simulink model "Sim_Riementrieb_2015a"  (R2015a)
settings: Solver=ode45  SolverMode=SingleTasking  StartTime=0.0  StopTime=20.0  RelTol=1e-3
InitFcn:
  | set_parameter
libraries: cstblocks x2
settings Model: Creator=wke  LastModifiedBy=Andreas
settings DataIOCC: SignalLoggingSaveFormat=ModelDataLogs
settings OptimizationCC: BlockReduction=off  BooleanDataType=off
settings DebuggingCC: SaveWithParameterizedLinksMsg=none  UnderspecifiedInitializationDetection=Classic  MergeDetectMultiDrivingBlocksExec=none  SignalResolutionControl=TryResolveAllWithWarning  MultiTaskDSMMsg=warning  MultiTaskCondExecSysMsg=none  StateNameClashWarn=warning
settings HardwareCC: TargetUnknown=on

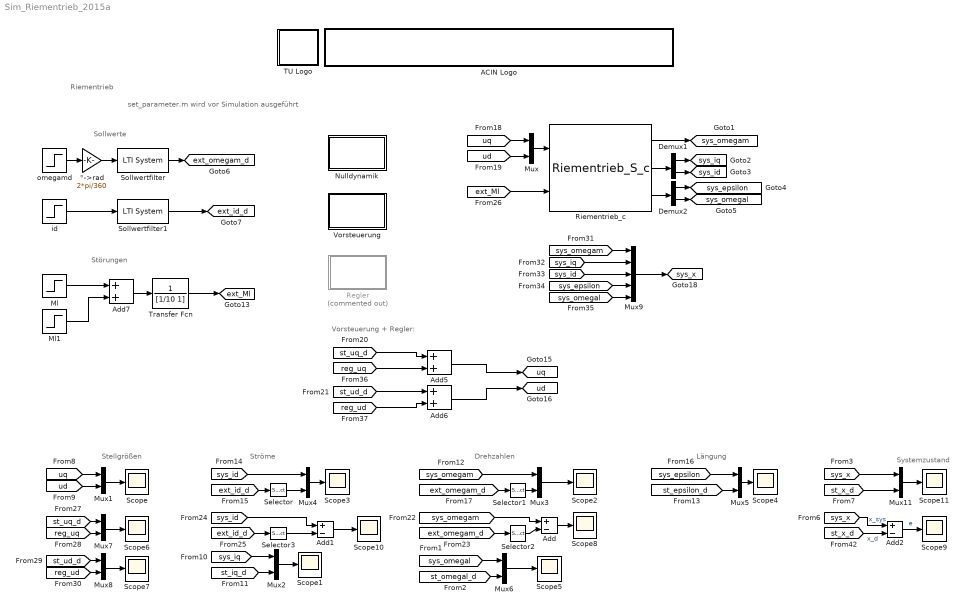
== system Sim_Riementrieb_2015a ==
  note: Vorsteuerung + Regler:
  note: Riementrieb
  note: set_parameter.m wird vor Simulation ausgeführt
  note: Sollwerte
  note: Stellgrößen
  note: Ströme
  note: Drehzahlen
  note: Längung
  note: Störungen
  note: Systemzustand
  ACIN Logo : Subsystem
      mask init:
      | s = get_param(gcb,'UserData');
      mask Display:
      | image(s.logo,[0 0 439 45]);
      | %axis image
  Add : Sum  Inputs=+-
  Add1 : Sum  Inputs=+-
  Add2 : Sum  Inputs=+-
  Add5 : Sum
  Add6 : Sum
  Add7 : Sum
  Demux1 : Demux  Outputs=2
  Demux2 : Demux  Outputs=2
  Ml : Step  Time=8  After=0.1  SampleTime=0
  Ml1 : Step  Time=15  After=-0.1  SampleTime=0
  Mux{,1..8,11} (10 alike) : Mux  Inputs=2
  Mux9 : Mux  Inputs=5
  Nulldynamik : Subsystem
  Regler : Subsystem  Commented=on
  Riementrieb_c : S-Function  FunctionName=Riementrieb_S_c  Parameters=parSys  SFunctionDeploymentMode=off  EnableBusSupport=off
      mask Display:
      | port_label('input',1,'uq,ud');
      | port_label('input',2,'Ml');
      | port_label('output',1,'omegam');
      | port_label('output',2,'iq,id');
      | port_label('output',3,'epsilon,omegal');
  Scope{,1..11} (12 alike) : Scope
      Scope settings: TimeRange=auto  ShowLegends=on  MaxDataPoints=5000  SaveToWorkspace=off  SaveName=ScopeData  YMin=3.34867  YMax=18.57408  SampleTime=-1
      Scope1 settings: TimeRange=auto  MaxDataPoints=5000  SaveToWorkspace=off  YMin=-300000  YMax=275000  SampleTime=-1
      Scope10 settings: TimeRange=auto  MaxDataPoints=5000  SaveToWorkspace=off  SaveName=ScopeData10  YMin=-10  YMax=10  SampleTime=-1
      Scope11 settings: TimeRange=auto  ShowLegends=on  MaxDataPoints=5000  SaveToWorkspace=off  SaveName=ScopeData11  YMin=-13.18283  YMax=118.51223  SampleTime=-1
      Scope2 settings: TimeRange=0.3051681706316654  ShowLegends=on  MaxDataPoints=5000  SaveToWorkspace=off  SaveName=ScopeData2  YMin=-13.53231  YMax=121.79079  SampleTime=-1
      Scope3 settings: TimeRange=1.762100082034454  MaxDataPoints=5000  SaveToWorkspace=off  SaveName=ScopeData3  YMin=-0.01741  YMax=0.15668  SampleTime=-1
      Scope4 settings: TimeRange=auto  MaxDataPoints=5000  SaveToWorkspace=off  SaveName=ScopeData4  YMin=-0.01592  YMax=0.00997  SampleTime=-1
      Scope5 settings: TimeRange=auto  MaxDataPoints=5000  SaveToWorkspace=off  SaveName=ScopeData5  YMin=-7.60944  YMax=68.48494  SampleTime=-1
      Scope6 settings: TimeRange=auto  MaxDataPoints=5000  SaveToWorkspace=off  SaveName=ScopeData6  YMin=-1.66533e-016  YMax=2.4  SampleTime=-1
      Scope7 settings: TimeRange=auto  MaxDataPoints=5000  SaveToWorkspace=off  SaveName=ScopeData7  YMin=-1.66533e-016  YMax=2.4  SampleTime=-1
      Scope8 settings: TimeRange=auto  MaxDataPoints=5000  SaveToWorkspace=off  SaveName=ScopeData8  YMin=-0.49523  YMax=3.98694  SampleTime=-1
      Scope9 settings: TimeRange=auto  ShowLegends=on  MaxDataPoints=5000  SaveToWorkspace=off  SaveName=ScopeData9  YMin=-7.00277  YMax=6.63987  SampleTime=-1
  Selector : Selector  InputPortWidth=2  IndexOptions=Index vector (dialog)  Indices=[1]  OutputSizes=1
  Selector1 : Selector  InputPortWidth=3  IndexOptions=Index vector (dialog)  Indices=[1]  OutputSizes=1
  Selector2 : Selector  InputPortWidth=3  IndexOptions=Index vector (dialog)  Indices=[1]  OutputSizes=1
  Selector3 : Selector  InputPortWidth=2  IndexOptions=Index vector (dialog)  Indices=[1]  OutputSizes=1
  Sollwertfilter : cstblocks/LTI System  sys=parReg.ssSF  IC=[]
  Sollwertfilter1 : cstblocks/LTI System  sys=parReg.ssSFi  IC=[]
  TU Logo : Subsystem
      mask init:
      | s = get_param(gcb,'UserData');
      mask Display: image(s.logo,[0 0 45 45]);
  Transfer Fcn : TransferFcn  Denominator=[1/10 1]
  Vorsteuerung : Subsystem
  id : Step  After=0.1  SampleTime=0
  omegamd : Step  Time=4  After=1000/60*360  SampleTime=0
  °->rad : Gain  Gain=2*pi/360
  tag scope: ext_Ml=global, ext_id_d=global, ext_omegam_d=global, sys_epsilon=global, sys_id=global, sys_iq=global, sys_omegal=global, sys_omegam=global, sys_x=global, ud=global, uq=global
  wires:
  Mux/1 -> Riementrieb_c/1
  °->rad/1 -> Sollwertfilter/1
  Sollwertfilter/1 -> [ext_omegam_d]
  Demux1/1 -> [sys_iq]
  Demux1/2 -> [sys_id]
  Demux2/1 -> [sys_epsilon]
  Demux2/2 -> [sys_omegal]
  Sollwertfilter1/1 -> [ext_id_d]
  id/1 -> Sollwertfilter1/1
  [uq] -> Mux1/1
  [ud] -> Mux1/2
  Mux1/1 -> Scope/1
  [sys_iq] -> Mux2/1
  [st_iq_d] -> Mux2/2
  Mux2/1 -> Scope1/1
  [sys_omegam] -> Mux3/1
  Mux3/1 -> Scope2/1
  [sys_id] -> Mux4/1
  [ext_id_d] -> Selector/1
  Mux4/1 -> Scope3/1
  [sys_epsilon] -> Mux5/1
  Mux5/1 -> Scope4/1
  [sys_omegal] -> Mux6/1
  Mux6/1 -> Scope5/1
  [ext_omegam_d] -> Selector1/1
  Selector1/1 -> Mux3/2
  Selector/1 -> Mux4/2
  [st_epsilon_d] -> Mux5/2
  [st_omegal_d] -> Mux6/2
  Add/1 -> Scope8/1
  [sys_omegam] -> Add/1
  [ext_omegam_d] -> Selector2/1
  Selector2/1 -> Add/2
  Add1/1 -> Scope10/1
  [sys_id] -> Add1/1
  [ext_id_d] -> Selector3/1
  Selector3/1 -> Add1/2
  omegamd/1 -> °->rad/1
  Transfer Fcn/1 -> [ext_Ml]
  [ext_Ml] -> Riementrieb_c/2
  [st_uq_d] -> Mux7/1
  [reg_uq] -> Mux7/2
  Mux7/1 -> Scope6/1
  [st_ud_d] -> Mux8/1
  [reg_ud] -> Mux8/2
  Mux8/1 -> Scope7/1
  Riementrieb_c/2 -> Demux1/1
  Riementrieb_c/3 -> Demux2/1
  Riementrieb_c/1 -> [sys_omegam]
  [sys_omegam] -> Mux9/1
  [sys_iq] -> Mux9/2
  [sys_id] -> Mux9/3
  [sys_epsilon] -> Mux9/4
  [sys_omegal] -> Mux9/5
  Mux9/1 -> [sys_x]
  Mux11/1 -> Scope11/1
  [sys_x] -> Mux11/1
  [st_x_d] -> Mux11/2
  [uq] -> Mux/1
  [ud] -> Mux/2
  Add2/1 -> Scope9/1  "e"
  [sys_x] -> Add2/1  "x_sys"
  [st_x_d] -> Add2/2  "x_d"
  [st_ud_d] -> Add6/1
  [reg_ud] -> Add6/2
  [reg_uq] -> Add5/2
  [st_uq_d] -> Add5/1
  Add5/1 -> [uq]
  Add6/1 -> [ud]
  Ml1/1 -> Add7/2
  Ml/1 -> Add7/1
  Add7/1 -> Transfer Fcn/1

== system Sim_Riementrieb_2015a/ACIN Logo ==

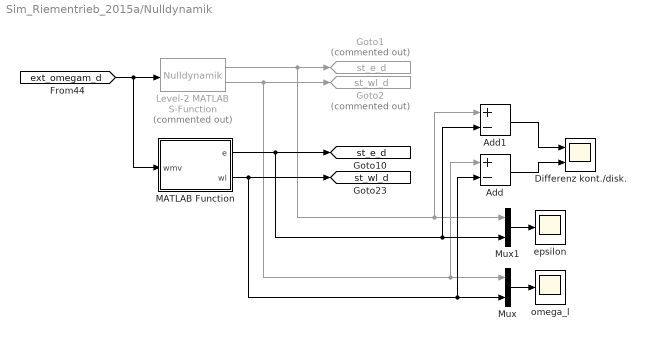
== system Sim_Riementrieb_2015a/Nulldynamik ==
  Add : Sum  Inputs=+-
  Add1 : Sum  Inputs=+-
  Differenz kont./disk. : Scope  NumInputPorts=2
      settings: TimeRange=auto  MaxDataPoints=5000  SaveToWorkspace=off  SaveName=ScopeData14  YMin=-0.000002~-0.00727  YMax=0.0000019~0.00518  SampleTime=-1
  Goto1 : Goto  Commented=on  GotoTag=st_e_d  TagVisibility=global
  Goto2 : Goto  Commented=on  GotoTag=st_wl_d  TagVisibility=global
  Level-2 MATLAB S-Function : M-S-Function  Commented=on  FunctionName=Nulldynamik  Parameters=parSys.eta_1_0 parSys.eta_2_0 [parSys.cr1 parSys.cr3 parSys.rl parSys.rm parSys.dl parSys.Il]
  MATLAB Function : MATLAB Function  TreatAsAtomicUnit=on
      settings: PermitHierarchicalResolution=ParametersOnly
  Mux : Mux  Inputs=2
  Mux1 : Mux  Inputs=2
  epsilon : Scope
      settings: TimeRange=auto  MaxDataPoints=5000  SaveToWorkspace=off  SaveName=ScopeData12  YMin=-0.014  YMax=0.008  SampleTime=-1
  omega_l : Scope
      settings: TimeRange=auto  MaxDataPoints=5000  SaveToWorkspace=off  SaveName=ScopeData13  YMin=-10  YMax=10  SampleTime=-1
  tag scope: st_e_d=global, st_wl_d=global
  wires:
  Level-2 MATLAB S-Function/1 -> Goto1/1, Add1/1, Mux1/1
  Level-2 MATLAB S-Function/2 -> Goto2/1, Add/1, Mux/1
  [ext_omegam_d] -> Level-2 MATLAB S-Function/1, MATLAB Function/1(wmv)
  MATLAB Function/1(e) -> [st_e_d], Add1/2, Mux1/2
  MATLAB Function/2(wl) -> [st_wl_d], Add/2, Mux/2
  Mux/1 -> omega_l/1
  Mux1/1 -> epsilon/1
  Add/1 -> Differenz kont./disk./2
  Add1/1 -> Differenz kont./disk./1

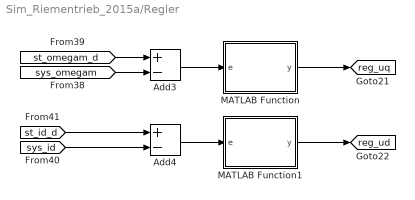
== system Sim_Riementrieb_2015a/Regler ==
  Add3 : Sum  Inputs=+-
  Add4 : Sum  Inputs=+-
  MATLAB Function : MATLAB Function  TreatAsAtomicUnit=on
      settings: PermitHierarchicalResolution=ParametersOnly
  MATLAB Function1 : MATLAB Function  TreatAsAtomicUnit=on
      settings: PermitHierarchicalResolution=ParametersOnly
  tag scope: reg_ud=global, reg_uq=global
  wires:
  MATLAB Function1/1(y) -> [reg_ud]
  Add3/1 -> MATLAB Function/1(e)
  Add4/1 -> MATLAB Function1/1(e)
  MATLAB Function/1(y) -> [reg_uq]
  [st_omegam_d] -> Add3/1
  [sys_id] -> Add4/2
  [sys_omegam] -> Add3/2
  [st_id_d] -> Add4/1

== system Sim_Riementrieb_2015a/TU Logo ==

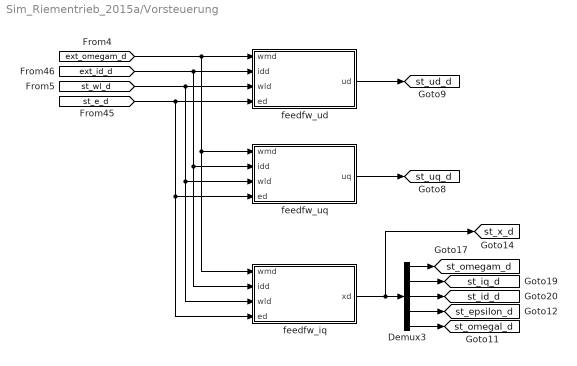
== system Sim_Riementrieb_2015a/Vorsteuerung ==
  Demux3 : Demux  Outputs=5
  feedfw_iq : MATLAB Function  TreatAsAtomicUnit=on
      settings: PermitHierarchicalResolution=ParametersOnly
  feedfw_ud : MATLAB Function  TreatAsAtomicUnit=on
      settings: PermitHierarchicalResolution=ParametersOnly
  feedfw_uq : MATLAB Function  TreatAsAtomicUnit=on
      settings: PermitHierarchicalResolution=ParametersOnly
  tag scope: st_epsilon_d=global, st_id_d=global, st_iq_d=global, st_omegal_d=global, st_omegam_d=global, st_ud_d=global, st_uq_d=global, st_x_d=global
  wires:
  feedfw_uq/1(uq) -> [st_uq_d]
  feedfw_iq/1(xd) -> [st_x_d], Demux3/1
  Demux3/4 -> [st_epsilon_d]
  Demux3/5 -> [st_omegal_d]
  Demux3/1 -> [st_omegam_d]
  Demux3/2 -> [st_iq_d]
  Demux3/3 -> [st_id_d]
  [ext_omegam_d] -> feedfw_iq/1(wmd), feedfw_uq/1(wmd), feedfw_ud/1(wmd)
  [st_wl_d] -> feedfw_iq/3(wld), feedfw_uq/3(wld), feedfw_ud/3(wld)
  [st_e_d] -> feedfw_iq/4(ed), feedfw_uq/4(ed), feedfw_ud/4(ed)
  feedfw_ud/1(ud) -> [st_ud_d]
  [ext_id_d] -> feedfw_iq/2(idd), feedfw_uq/2(idd), feedfw_ud/2(idd)

== matlab function Sim_Riementrieb_2015a/Vorsteuerung/feedfw_ud ==
  data: wmd input; idd input; ud output; wld input; ed input; parSys parameter
function ud  = feedfw_ud(wmd, idd, wld, ed, parSys)
%#codegen
wm = wmd(1);
wmp = wmd(2);
wmpp = wmd(3);
id = idd(1);
idp = idd(2);
wl = wld;
e = ed;

%parameter;
%Zuweisungen
Lm = parSys.Lm;
Rm = parSys.Rm;
cr1 = parSys.cr1;
cr3 = parSys.cr3;
rm = parSys.rm;
dm = parSys.dm;
rl = parSys.rl;
dl = parSys.dl;
I_l = parSys.Il;
I_m = parSys.Im;
p = parSys.p;
Phi = parSys.Phi;

iq = 0.2e1 / 0.3e1 * (-2 * cr3 * e ^ 3 * rm - 2 * cr1 * e * rm + wmp * I_m + dm * wm) / Phi / p;
ud = 0.3e1 / 0.2e1 * Lm * p * wm * iq + 0.3e1 / 0.2e1 * idp * Lm + Rm * id;


end

== matlab function Sim_Riementrieb_2015a/Nulldynamik/MATLAB Function ==
  settings: updateMethod=DISCRETE  sampleTime=parSys.TsID
  data: wmv input; e output; wl output; parSys parameter
function [e, wl] = Null_disc(wmv, parSys)
%#codegen
persistent k
persistent x1 % epsilon
persistent x2 % omega_l
persistent wm_old

wm = wmv(1);


if (isempty(k))
    k = 0;
end
if (isempty(x1))
    x1 = parSys.eta_1_0;
end
if (isempty(x2))
    x2 = parSys.eta_2_0;
end
if (isempty(wm_old))
    wm_old = 0;
end

cr1 = parSys.cr1;
cr3 = parSys.cr3;
Il = parSys.Il;
rl = parSys.rl;
rm = parSys.rm;
dl = parSys.dl;

% explizites Heun-Verfahren
k = k + parSys.TsID;

f1 = rl*x2-rm*wm_old; % epsilon
f2 = 1/Il*(-2*(cr1*x1+cr3*x1^3)*rl - dl*x2); % omega_l

xp1 = x1 + parSys.TsID*f1;
xp2 = x2 + parSys.TsID*f2;

x1 = x1 + parSys.TsID/2*(f1 + (rl*xp2 - rm*wm));
x2  = x2 + parSys.TsID/2*(f2 + 1/Il*(-2*(cr1*xp1 + cr3*xp1^3)*rl - dl*xp2));

e = x1;
wl = x2;

wm_old = wm;
end

== matlab function Sim_Riementrieb_2015a/Vorsteuerung/feedfw_uq ==
  data: wmd input; idd input; uq output; wld input; ed input; parSys parameter
function uq  = feedfw_uq(wmd, idd, wld, ed, parSys)
%#codegen
wm = wmd(1);
wmp = wmd(2);
wmpp = wmd(3);
id = idd(1);
idp = idd(2);
wl = wld;
e = ed;

%parameter;
%Zuweisungen
Lm = parSys.Lm;
Rm = parSys.Rm;
cr1 = parSys.cr1;
cr3 = parSys.cr3;
rm = parSys.rm;
dm = parSys.dm;
rl = parSys.rl;
dl = parSys.dl;
I_l = parSys.Il;
I_m = parSys.Im;
p = parSys.p;
Phi = parSys.Phi;

iq = 0.2e1 / 0.3e1 * (-2 * cr3 * e ^ 3 * rm - 2 * cr1 * e * rm + wmp * I_m + dm * wm) / Phi / p;
uq = Lm * I_m / Phi / p * (wmpp + 0.1e1 / I_m ^ 2 * dm * ((2 * (cr3 * e ^ 3 + cr1 * e) * rm) - dm * wm + 0.3e1 / 0.2e1 * Phi * p * iq) - 0.1e1 / I_m * Phi * p / Lm * (-Rm * iq + 0.3e1 / 0.2e1 * Lm * p * wm * id - Phi * p * wm) - 0.2e1 / I_m * (3 * cr3 * e ^ 2 + cr1) * rm * (rl * wl - rm * wm));


end

== matlab function Sim_Riementrieb_2015a/Vorsteuerung/feedfw_iq ==
  data: wmd input; idd input; xd output; wld input; ed input; parSys parameter
function xd  = feedfw_iq(wmd, idd, wld, ed, parSys)
%#codegen
wm = wmd(1);
wmp = wmd(2);
wmpp = wmd(3);
id = idd(1);
idp = idd(2);
wl = wld;
e = ed;

%parameter;
%Zuweisungen
Lm = parSys.Lm;
Rm = parSys.Rm;
cr1 = parSys.cr1;
cr3 = parSys.cr3;
rm = parSys.rm;
dm = parSys.dm;
rl = parSys.rl;
dl = parSys.dl;
I_l = parSys.Il;
I_m = parSys.Im;
p = parSys.p;
Phi = parSys.Phi;

iq = 0.2e1 / 0.3e1 * (-2 * cr3 * e ^ 3 * rm - 2 * cr1 * e * rm + wmp * I_m + dm * wm) / Phi / p;

xd = [wm iq id e wl];


end

== matlab function Sim_Riementrieb_2015a/Regler/MATLAB Function ==
  settings: updateMethod=DISCRETE  sampleTime=0.1e-3
  data: e input; y output; parPI parameter
function y = fcn(e, parPI)
%#codegen
persistent x
if (isempty(x))
    x = 0;
end

x = parPI.a2*x+parPI.b2*e;
y = parPI.c2*x+parPI.d2*e;

end

== matlab function Sim_Riementrieb_2015a/Regler/MATLAB Function1 ==
  settings: updateMethod=DISCRETE  sampleTime=0.1e-3
  data: e input; y output; parPI parameter
function y = fcn(e, parPI)
%#codegen
persistent x
if (isempty(x))
    x = 0;
end

x = parPI.a1*x+parPI.b1*e;
y = parPI.c1*x+parPI.d1*e;

end
